simulink model "Solar_Powered_Sucker_Rod_Pump_Final_Publish_Default_Summer"  (R2024a)
settings: Solver=ode23t  StartTime=0.0  StopTime=19  RelTol=1e-3
undefined symbols (not defined in the file or in its folder): Acid, Lead, sigbuilder_block
libraries: spsVoltageMeasurementLib x4, spsSeriesRLCBranchLib x3, spsCurrentMeasurementLib x2, spsAsynchronousMachinepuUnitsLib x1, spsBatteryLib x1, spsDiodeLib x1, spsMosfetLib x1, spsPVArrayLib x1, spsPWMGenerator2LevelLib x1, spsPWMGeneratorDCDCLib x1, eePowerMeasurement x1, spsThreePhaseTransformerTwoWindingsLib x1
settings Model: Creator=Dell  LastModifiedBy=USER
settings SolverCC: AlgebraicLoopSolver=TrustRegion
settings DebuggingCC: UnconnectedInputMsg=warning  UnconnectedOutputMsg=warning  UnconnectedLineMsg=warning
settings ModelReferenceCC: EnableRefExpFcnMdlSchedulingChecks=on
settings RTWCC: GPUComputeCapability=3.5  DLArmComputeVersion=19.05

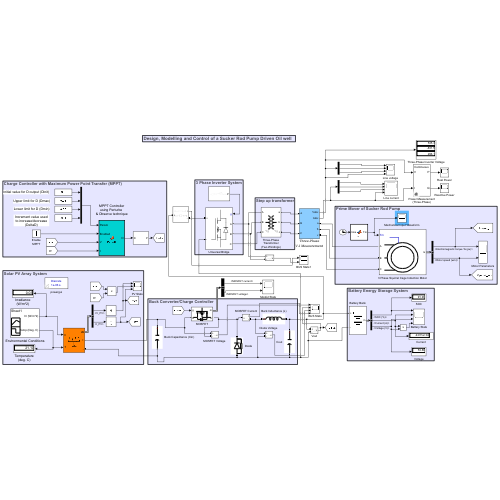
[thumbnail: Simulink's stored preview of the top-level diagram]
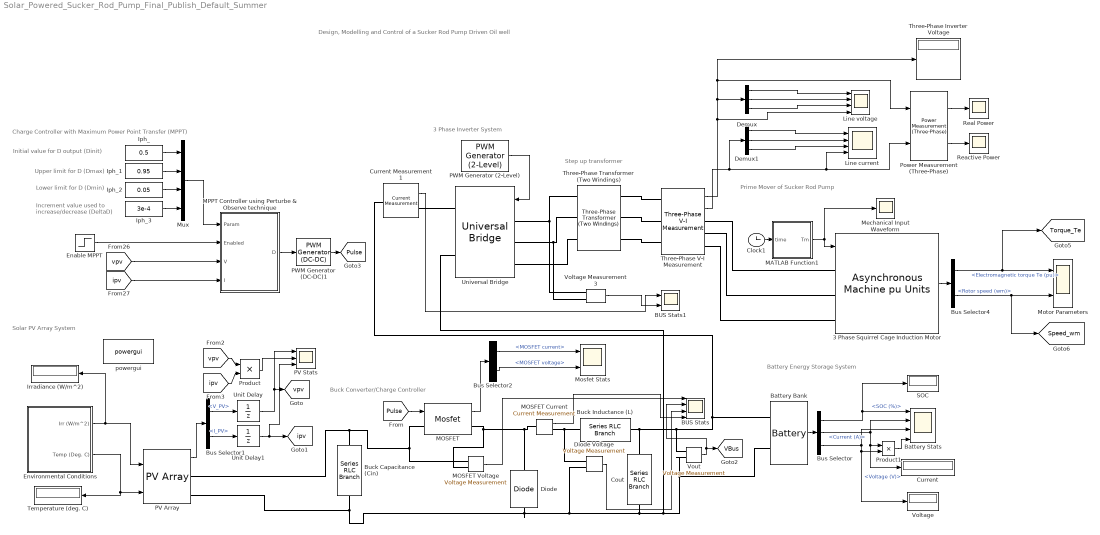
== system Solar_Powered_Sucker_Rod_Pump_Final_Publish_Default_Summer ==
  note: Design, Modelling and Control of a Sucker Rod Pump Driven Oil well
  note: Step up transformer
  note: Solar PV Array System
  note: Prime Mover of Sucker Rod Pump
  note: Battery Energy Storage System
  note: Buck Converter/Charge Controller
  note: Charge Controller with Maximum Power Point Transfer (MPPT)
  note: Lower limit for D (Dmin)
  note: Increment value used to increase/decrease (DeltaD)
  note: Upper limit for D (Dmax)
  note: Initial value for D output (Dinit)
  note: 3 Phase Inverter System
  " MOSFET Current " : spsCurrentMeasurementLib/Current Measurement  PhasorSimulation=off  OutputType=Complex  PSBequivalent=0
  3 Phase Squirrel Cage Induction Motor : spsAsynchronousMachinepuUnitsLib/Asynchronous Machine pu Units  RotorType=Squirrel-cage  PresetModel=No  MechanicalLoad=Torque Tm  ShowDetailedParameters=on  ReferenceFrame=Rotor  Units=pu  MeasurementBus=off  NominalParameters=[4670 460 60]  VoltageRatio=1  Stator=[0.09002 0.01367]  Rotor=[0.01909 0.0397]  Cage1=[0.07147 0.01399]  Cage2=[0.07178 0.01367]  Lm=1.051  Mechanical=[0.09526 0.05479 3]  PolePairs=2  InitialConditions=[0.03 0 0.8,-0.4,-0.4 0,-120,120]  SimulateSaturation=off  Saturation="[0.212,0.4201,0.8125,1.0979,1.4799,2.2457,3.2586,4.5763,6.4763 ;   0.5,0.7,0.9,1,1.1,1.2 ,1.3,1.4,1.5]"  LoadFlowParameters=0  TsPowergui=0  TsBlock=1e-6  IterativeModel=Trapezoidal non iterative  IterativeDiscreteModel=Backward Euler robust  Pmec=4.44e3
      settings: LibrarySourceBlock=|
      | sps_lib/Electrical Machines/Asynchronous Machine
      | pu Units
  BUS Stats : Scope  NumInputPorts=4
  BUS Stats1 : Scope  NumInputPorts=2
  Battery Bank : spsBatteryLib/Battery  BatType=Lead-Acid  ShowTempParam=off  ThermalPreset=no  ShowAgeParam=off  NomV=48  NomQ=3504  SOC=75  Batt_Tr=1e-6  PresetModel=on  MaxQ=3650  MinV=36  FullV=52.2632  Dis_rate=700.8  R=0.00013699  Normal_OP=1087.2133  expZone="[48.8684        11.68]"  current=[6.5 13 32.5]  Units=Time  Tci=20  NomT=20  T2=-30  MaxQ2=4.8  FullV2=7.1  Normal_OP2=5.655  expZone2="[6.58           1]"  Rca=0.6  ti=2000  Dp=0  Neq0=0  Tsim=1e6  Ta1=25  Qeol=5.4*0.9  Reol=0.013333*1.2  Char_age=[2.3478, 3]  Dis_age=[2.3478, 10]  N1=1500  N2=10500  N3=1000  N4=1400  Ta2=45  N5=950
      settings: LibrarySourceBlock=electricdrivelib/Extra Sources/Battery
  Battery Stats : Scope  NumInputPorts=4
  Buck Capacitance (Cin) : spsSeriesRLCBranchLib/Series RLC Branch  LConnTagsString=__new0  RConnTagsString=__new0  BranchType=C  Resistance=0.001  Inductance=1e-3  SetiL0=off  InitialCurrent=0  Capacitance=4740e-6  Setx0=off  InitialVoltage=0  Measurements=None
  Buck Inductance (L) : spsSeriesRLCBranchLib/Series RLC Branch  LConnTagsString=__new0  RConnTagsString=__new0  BranchType=L  Resistance=1  Inductance=17.319e-6  SetiL0=off  InitialCurrent=0  Capacitance=1e-6  Setx0=off  InitialVoltage=0  Measurements=None
  Bus Selector : BusSelector  OutputSignals=SOC (%),Current (A),Voltage (V)
  Bus Selector1 : BusSelector  OutputSignals=V_PV,I_PV
  Bus Selector2 : BusSelector  OutputSignals=MOSFET current,MOSFET voltage
  Bus Selector4 : BusSelector  OutputSignals=Mechanical.Electromagnetic torque Te (pu),Mechanical.Rotor speed (wm)
  Clock1 : Clock
      settings: Decimation=19
  Cout : spsSeriesRLCBranchLib/Series RLC Branch  LConnTagsString=__new0  RConnTagsString=__new0  BranchType=C  Resistance=1  Inductance=369.79e-6  SetiL0=off  InitialCurrent=0  Capacitance=5924.48e-6  Setx0=off  InitialVoltage=0  Measurements=None
  Current : Display
  Current Measurement1 : spsCurrentMeasurementLib/Current Measurement  PhasorSimulation=off  OutputType=Complex  PSBequivalent=0
  Demux : Demux  Outputs=3
  Demux1 : Demux  Outputs=3
  Diode : spsDiodeLib/Diode  Ron=0.001  Lon=0  Vf=0.8  IC=0  UseSnubber=0  Rs=500  Cs=250e-9  Measurements=off
  "Diode Voltage " : spsVoltageMeasurementLib/Voltage Measurement  PhasorSimulation=off  OutputType=Complex  PSBequivalent=0
  Enable MPPT : Step  Time=0.002  SampleTime=0
  Environmental Conditions : Subsystem  Tag=STV Subsys  LoadFcn=sigbuilder_block('load',[224.25 144.75 303 314.25 ]);  StartFcn=sigbuilder_block('start');  StopFcn=sigbuilder_block('stop');  ClipboardFcn=sigbuilder_block('clipboard');  mask(Sigbuilder block){tuvar=[0:10]}
      mask help: Sigbuilder GUI
      mask init:
      | if ~strcmp(get_param(bdroot(gcbh),'SimulationStatus'),'stopped') tuvar = sigbuilder_block('maskInit'); end
      settings: CopyFcn=sigbuilder_block('copy');  DeleteFcn=sigbuilder_block('delete');  ModelCloseFcn=sigbuilder_block('modelClose');  PreSaveFcn=sigbuilder_block('preSave');  PauseFcn=sigbuilder_block('pause')  ContinueFcn=sigbuilder_block('continue')  NameChangeFcn=sigbuilder_block('namechange');  OpenFcn=sigbuilder_block('open',[224.25 144.75 550.5 354.75 ]);  CloseFcn=sigbuilder_block('close');
      mask Display: plot(0, 0, 100, 100,[2, 2, 32, 32, 2], [68, 8, 8, 68, 68],[32, 2], [38, 38], [32, 19, 2],[53, 60, 44], [32, 17, 17, 2],[16, 16, 31, 31]);txt = getActiveGroup(gcbh);text(2, 100, txt,'verticalAlignment', 'top');
  Iph_ : Constant  Value=0.5
  Iph_1 : Constant  Value=0.95
  Iph_2 : Constant  Value=0.05
  Iph_3 : Constant  Value=3e-4
  Irradiance (W/m^2) : Display
      settings: Format=bank  Decimation=1000
  Line current : Scope  NumInputPorts=4
  Line voltage : Scope  NumInputPorts=4
  MATLAB Function1 : MATLAB Function  TreatAsAtomicUnit=on
  MOSFET : spsMosfetLib/Mosfet  Ron=0.1  Lon=0  Rd=0.01  Vfd=0  IC=0  Rs=1e5  Cs=inf  Measurements=on
  "MOSFET Voltage " : spsVoltageMeasurementLib/Voltage Measurement  PhasorSimulation=off  OutputType=Complex  PSBequivalent=0
  "MPPT Controller using Perturbe & Observe technique " : MATLAB Function  TreatAsAtomicUnit=on
  Mechanical Input Waveform : Scope
  Mosfet Stats : Scope  NumInputPorts=2
  Motor Parameters : Scope  NumInputPorts=2
  Mux : Mux
  PV Array : spsPVArrayLib/PV Array  Npar=46  Nser=2  PlotType=array @ 1000 W/m2 & specified temperatures  S_vec="[ 1000  500  100 ]"  Temp_C_vec="[ 45 25  ]"  ModuleName=Jinko Solar Co._ Ltd JKM300M-60  PlotWhenSelected=off  Pm=300.246  Ncell=60  Voc=40.1  Isc=9.72  Vm=32.6  Im=9.21  beta_Voc_pc=-0.308  alpha_Isc_pc=0.065  beta_Voc=-0.12351  alpha_Isc=0.006318  IL=9.7474  I0=4.7373e-11  nI=0.99895  Rsh=437.5209  Rs=0.31013  RobustModel=off  RobustCellTemperature=313.3991  BAL=on  Tc=1e-6  Tfilter=5e-5
  PV Stats : Scope  NumInputPorts=3
  PWM Generator (2-Level) : spsPWMGenerator2LevelLib/PWM Generator (2-Level)  ModulatorType=Three-phase bridge (6 pulses)  ModulatorMode=Unsynchronized  Fc=27*60  Pc=90  nF=27  MinMax="[ -1  1 ]"  SamplingTechnique=Natural  ModulatingSignals=on  m=0.8  Freq=60  Phase=0  Ts=1e-6  ShowCarrierOutport=off
  PWM Generator (DC-DC)1 : spsPWMGeneratorDCDCLib/PWM Generator (DC-DC)  Fsw=5000  Ts=1e-6
  Power Measurement (Three-Phase) : eePowerMeasurement/Power Measurement (Three-Phase)  LabelModeActiveChoice=Continuous  F=60  K=[0 1 2 3]  Seq=Positive  Ts=0
  Product : Product
  Product1 : Product
  Reactive Power : Scope
  Real Power : Scope
  SOC : Display
  Temperature (deg. C) : Display
      settings: Format=bank  Decimation=1000
  Three-Phase Transformer (Two Windings) : spsThreePhaseTransformerTwoWindingsLib/Three-Phase Transformer (Two Windings)  Winding1Connection=Yg  Winding2Connection=Yg  CoreType=Three single-phase transformers  SetSaturation=off  Hysteresis=off  DataFile='hysteresis'  SetInitialFlux=off  Measurements=None  UNITS=SI  NominalPower=[ 7e3 , 60 ]  Winding1=[24 0.00025714 2.7284e-05]  Winding2=[460 0.060457 0.0064147]  Rm=64.286  Lm=0.17052  L0=0.5  Saturation=[0 0;0.45724 0.07797;190.52 0.098762]  InitialFluxes=[ 0.8 , -0.8 , 0.7 ]  BreakLoop=off  DiscreteSolver=Backward Euler robust  DataType=on  TransfoNumber=1
  Three-Phase V-I Measurement : spsThreePhaseVIMeasurementLib/Three-Phase V-I Measurement  VoltageMeasurement=phase-to-phase  SetLabelV=off  LabelV=Vabc  Vpu=off  VpuLL=off  CurrentMeasurement=yes  SetLabelI=off  LabelI=Iabc  Ipu=off  Pbase=100e6  Vbase=500e3  OutputType=Complex  PhasorSimulation=off  PSBequivalent=0
  Three-Phase Inverter Voltage : Display
  Unit Delay : UnitDelay  SampleTime=1e-4  HasFrameUpgradeWarning=on
  Unit Delay1 : UnitDelay  SampleTime=1e-4  HasFrameUpgradeWarning=on
  Universal Bridge : spsUniversalBridgeLib/Universal Bridge  Arms=3  SnubberResistance=1e5  SnubberCapacitance=inf  Device=MOSFET / Diodes  Ron=1e-3  Lon=0  ForwardVoltages="[  0  0  ]"  ForwardVoltage=0  GTOparameters=[ 10e-6 , 20e-6 ]  IGBTparameters=[ 1e-6 , 2e-6 ]  Measurements=None  Measurements_2=None  converterType=Rectifier
  Voltage : Display
  Voltage Measurement3 : spsVoltageMeasurementLib/Voltage Measurement  PhasorSimulation=off  OutputType=Complex  PSBequivalent=0
  Vout : spsVoltageMeasurementLib/Voltage Measurement  PhasorSimulation=off  OutputType=Complex  PSBequivalent=0
  powergui : spspowerguiLib/powergui  Priority=1  SimulationMode=Discrete  SampleTime=1e-6  frequency=60  Iterations=50  frequencyindice=0  Pbase=100e6  ErrMax=1e-4  UnitsV=kV  UnitsW=MW  buscounter=0  FunctionMessages=off  echomessages=off  EnableUseOfTLC=off  CurrentSourceSwitches=off  DisableSnubberDevices=off  DisableRonSwitches=off  DisableVfSwitches=off  DisplayEquations=off  AutomaticDiscreteSolvers=off  SolverType=Tustin/Backward Euler (TBE)  Interpol=off  ExternalGateDelay=off  methode=off  Ts=100  x0status=blocks  SPID=on  SwTol=0  HookPort=off  NonlinearTolerance=1e-4  nMaxIteration=100  ContinueOnMaxIteration=off  RestoreLinks=warning  ResistiveCurrentMeasurement=off  Frange=[0:2:500]  Ylog=off  Xlog=on  ShowGrid=off  save=off  variable=ZData  structure=0  ZoomFFT=off  StartTime=0.0  cycles=1  DisplayStyle=1  fundamental=60  FreqAxis=off  MaxFrequency=1000  frequencyindicesteady=1  RmsSteady=1  display=off
  tag scope: Pulse=global, Speed_wm=global, Torque_Te=global, VBus=global, ipv=global, vpv=global
  wires:
  Battery Bank/1 -> Bus Selector/1
  Bus Selector/1 -> Battery Stats/1, SOC/1  "<SOC (%)>"
  Bus Selector/3 -> Battery Stats/3, Voltage/1, Product1/2  "<Voltage (V)>"
  Bus Selector/2 -> Battery Stats/2, Current/1, Product1/1  "<Current (A)>"
  PV Array/1 -> Bus Selector1/1
  Bus Selector1/1 -> Unit Delay/1  "<V_PV>"
  Bus Selector1/2 -> Unit Delay1/1  "<I_PV>"
  Unit Delay/1 -> PV Stats/1, [vpv]
  Unit Delay1/1 -> PV Stats/3, [ipv]
  [vpv] -> Product/1
  [ipv] -> Product/2
  Product/1 -> PV Stats/2
  "MPPT Controller using Perturbe & Observe technique "/1(D) -> PWM Generator (DC-DC)1/1
  Iph_1/1 -> Mux/2
  Iph_/1 -> Mux/1
  [vpv] -> "MPPT Controller using Perturbe & Observe technique "/3(V)
  Mux/1 -> "MPPT Controller using Perturbe & Observe technique "/1(Param)
  Iph_2/1 -> Mux/3
  Iph_3/1 -> Mux/4
  [ipv] -> "MPPT Controller using Perturbe & Observe technique "/4(I)
  Enable MPPT/1 -> "MPPT Controller using Perturbe & Observe technique "/2(Enabled)
  PWM Generator (DC-DC)1/1 -> [Pulse]
  MOSFET/1 -> Bus Selector2/1
  Bus Selector2/1 -> Mosfet Stats/1  "<MOSFET current>"
  Bus Selector2/2 -> Mosfet Stats/2  "<MOSFET voltage>"
  Vout/1 -> [VBus], BUS Stats/2
  "MOSFET Voltage "/1 -> BUS Stats/1
  "Diode Voltage "/1 -> BUS Stats/3
  " MOSFET Current "/1 -> BUS Stats/4
  [Pulse] -> MOSFET/1
  PWM Generator (2-Level)/1 -> Universal Bridge/1
  Current Measurement1/1 -> BUS Stats1/1
  Voltage Measurement3/1 -> BUS Stats1/2
  Demux1/1 -> Line current/1
  Demux1/2 -> Line current/2
  Demux/1 -> Line voltage/1
  Demux/2 -> Line voltage/2
  Power Measurement (Three-Phase)/1 -> Real Power/1
  Demux1/3 -> Line current/3
  Power Measurement (Three-Phase)/2 -> Reactive Power/1
  Demux/3 -> Line voltage/3
  Bus Selector4/2 -> [Speed_wm], Motor Parameters/2  "<Rotor speed (wm)>"
  Bus Selector4/1 -> [Torque_Te], Motor Parameters/1  "<Electromagnetic torque Te (pu)>"
  Clock1/1 -> MATLAB Function1/1(time)
  Three-Phase V-I Measurement/2 -> Demux1/1, Line current/4, Power Measurement (Three-Phase)/2
  3 Phase Squirrel Cage Induction Motor/1 -> Bus Selector4/1
  Three-Phase V-I Measurement/1 -> Line voltage/4, Three-Phase Inverter Voltage/1, Power Measurement (Three-Phase)/1, Demux/1
  MATLAB Function1/1(Tm) -> 3 Phase Squirrel Cage Induction Motor/1, Mechanical Input Waveform/1
  Product1/1 -> Battery Stats/4
  Environmental Conditions/1(Irr (W/m^2)) -> PV Array/1, Irradiance (W/m^2)/1
  Environmental Conditions/2(Temp (Deg. C)) -> Temperature (deg. C)/1, PV Array/2
  connections:
  Buck Capacitance (Cin)/LConn1 -- "MOSFET Voltage "/LConn1 -- MOSFET/LConn1 -- PV Array/RConn1
  PV Array/RConn2 -- Battery Bank/LConn2 -- Vout/LConn2 -- Universal Bridge/RConn2 -- Cout/RConn1 -- "Diode Voltage "/LConn2 -- Diode/LConn1 -- Buck Capacitance (Cin)/RConn1
  Diode/RConn1 -- " MOSFET Current "/LConn1 -- "MOSFET Voltage "/LConn2 -- MOSFET/RConn1
  Cout/LConn1 -- Battery Bank/LConn1 -- Current Measurement1/LConn1 -- Vout/LConn1 -- Buck Inductance (L)/RConn1
  Buck Inductance (L)/LConn1 -- " MOSFET Current "/RConn1 -- "Diode Voltage "/LConn1
  Three-Phase Transformer (Two Windings)/LConn1 -- Voltage Measurement3/LConn1 -- Universal Bridge/LConn1
  Universal Bridge/LConn3 -- Three-Phase Transformer (Two Windings)/LConn3
  Universal Bridge/LConn2 -- Three-Phase Transformer (Two Windings)/LConn2 -- Voltage Measurement3/LConn2
  Universal Bridge/RConn1 -- Current Measurement1/RConn1
  Three-Phase V-I Measurement/RConn1 -- 3 Phase Squirrel Cage Induction Motor/LConn1
  Three-Phase V-I Measurement/RConn3 -- 3 Phase Squirrel Cage Induction Motor/LConn3
  Three-Phase V-I Measurement/RConn2 -- 3 Phase Squirrel Cage Induction Motor/LConn2
  Three-Phase V-I Measurement/LConn2 -- Three-Phase Transformer (Two Windings)/RConn2
  Three-Phase Transformer (Two Windings)/RConn3 -- Three-Phase V-I Measurement/LConn3
  Three-Phase V-I Measurement/LConn1 -- Three-Phase Transformer (Two Windings)/RConn1

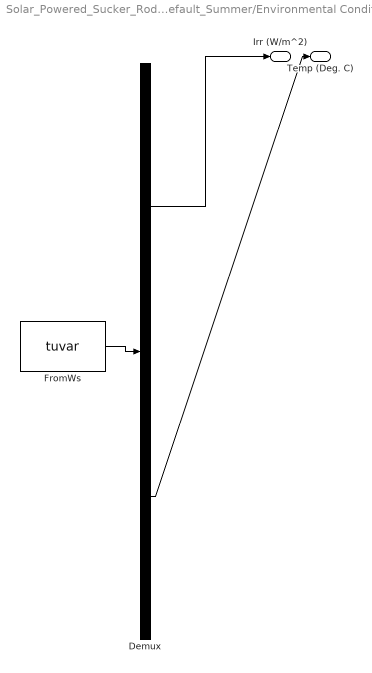
== system Solar_Powered_Sucker_Rod_Pump_Final_Publish_Default_Summer/Environmental Conditions ==
  Demux : Demux  Tag=STV Demux  Outputs=2
      settings: DisplayOption=none
  FromWs : FromWorkspace  Tag=STV FromWs  VariableName=tuvar
      SigBuilderData=|
      | common.afterFinalStr = 'Extrapolate'
      | common.sampleTime = '0'
      | dataSet.timeRange = [1 19]
      | dataSet.name = 'Sheet1'
      | sbobj.Groups.Name = 'Sheet1'
      | sbobj.Groups.Signals(1).Name = 'Irr (W/m^2)'
      | sbobj.Groups.Signals(1).XData = [1 2 3 4 5 6 7 8 9 10 11 12 13 14 15 16 17 18 19]
      | sbobj.Groups.Signals(1).YData = [0 138.4 784.7 1513.4 2236.23333333 2904.33333333 3471.8 3899.9 4160.3 4233.5 4116.66666667 3816.63333333 3353.83333333 2759.93333333 2075.26666667 1346.56666667 623.966666667 59.7666666667 0]
      | sbobj.Groups.Signals(2).Name = 'Temp (Deg. C)'
      | sbobj.Groups.Signals(2).XData = [1 2 3 4 5 6 7 8 9 10 11 12 13 14 15 16 17 18 19]
      | sbobj.Groups.Signals(2).YData = [9.6 9.7 9.9 11.7 15.3 19 21.5 22.9 24.7 25 24.6 27.3 26.9 27.1 27.4 27 26 23.8 21.1]
      | sbobj.Groups.TimeRange = [1 19]
  Irr (W/m^2) : Outport  Tag=STV Outport  VectorParamsAs1DForOutWhenUnconnected=off
  Temp (Deg. C) : Outport  Tag=STV Outport  Port=2
  wires:
  Demux/1 -> Irr (W/m^2)/1
  FromWs/1 -> Demux/1
  Demux/2 -> Temp (Deg. C)/1

== matlab function Solar_Powered_Sucker_Rod_Pump_Final_Publish_Default_Summer/MATLAB Function1 ==
  data: time input; Tm output
function Tm = fcn(time)
    % Define base values for 6-pole motor
    base_power = 4670;    % W
    base_speed = 1200;   % rad/s (synchronous speed for 3-pole motor at 60 Hz)
    base_torque = base_power/base_speed;  % Base torque ≈ 3.9 N⋅m

    % Define parameters for the pump torque profile in per unit
    params.base_torque = 0.8;        % 80% of rated torque
    params.torque_amplitude = 0.2;    % 20% torque variation
    params.pump_freq = 0.2;          % Pump frequency (Hz)
    params.phase = 0;                % Initial phase (radians)

    % Calculate varying torque in per unit
    Tm = params.base_torque + ...
         params.torque_amplitude * sin(2*pi*params.pump_freq*time + params.phase);

    % Add higher frequency components (also in per unit)
    harmonic2 = 0.3 * params.torque_amplitude * sin(4*pi*params.pump_freq*time);
    harmonic3 = 0.2 * params.torque_amplitude * sin(6*pi*params.pump_freq*time);
    Tm = Tm + harmonic2 + harmonic3;

    % Ensure torque doesn't go below minimum value (0.2 pu)
    min_torque = 0.2;
    Tm = max(Tm, min_torque);
    
    % For debugging purposes, uncomment to see actual torque values
    % Tm = Tm * base_torque;  % This would give torque in N⋅m
end

== matlab function Solar_Powered_Sucker_Rod_Pump_Final_Publish_Default_Summer/MPPT Controller using Perturbe & Observe technique  ==
  settings: updateMethod=DISCRETE  sampleTime=Ts_Control
  data: Param input; Enabled input; V input; I input; D output
function D = PandO(Param, Enabled, V, I)
    % MPPT controller based on the Perturb & Observe algorithm.
    % D output = Duty cycle of the boost converter (value between 0 and 1)
    %
    % Inputs:
    %   Param: Array containing [Dinit, Dmax, Dmin, deltaD]
    %   Enabled: Flag to enable the MPPT controller (1 = enabled)
    %   V: PV array terminal voltage (V)
    %   I: PV array current (A)
    
    % Parameters from input
    Dinit = Param(1);  % Initial value for D output
    Dmax = Param(2);   % Maximum value for D
    Dmin = Param(3);   % Minimum value for D
    deltaD = Param(4); % Increment value used to adjust the duty cycle D
    
    % Persistent variables to store previous values
    persistent Vold Pold Dold;
    
    if isempty(Vold)
        Vold = 0;
        Pold = 0;
        Dold = Dinit;
    end
    
    % Calculate current power and changes in voltage and power
    P = V * I;
    dV = V - Vold;
    dP = P - Pold;
    
    % Adjust duty cycle based on changes in power and voltage
    if abs(dP) > 1e-9 && Enabled ~= 0
        if dP < 0
            if dV < 0
                D = Dold - deltaD;
            else
                D = Dold + deltaD;
            end
        else
            if dV < 0
                D = Dold + deltaD;
            else
                D = Dold - deltaD;
            end    
        end
    else
        D = Dold;
    end
    
    % Ensure duty cycle stays within specified limits
    if D > Dmax || D < Dmin
        D = max(min(D, Dmax), Dmin);
    end
    
    % Update persistent variables for next iteration
    Dold = D;
    Vold = V;
    Pold = P;
end
